simulink model "SVPWMtrials"  (R2015b)
settings: Solver=VariableStepAuto  StartTime=0.0  StopTime=1  RelTol=1e-3
libraries: powerlib x25
(part 3 of 3)

== matlab function SVPWMtrials/Sector2 ==
  data: Sector2 input; Sa1 output; Sa2 output; Sa1P output; Sa2P output; Sb1 output; Sb2 output; Sb1P output; Sb2P output; Sc1 output; Sc2 output; Sc1P output; Sc2P output; rgn2a input; rgn2b input; rgn3 input; rgn4 input; exttime input; Ta input; Tb input; Tc input
function [Sa1, Sa2, Sa1P, Sa2P, Sb1, Sb2, Sb1P, Sb2P, Sc1, Sc2, Sc1P, Sc2P] = fcn(Sector2,rgn2a, rgn2b, rgn3, rgn4,exttime, Ta, Tb, Tc)

Sa1=0; Sa2=0; Sa1P=0; Sa2P=0; Sb1=0; Sb2=0; Sb1P=0; Sb2P=0; Sc1=0; Sc2=0; Sc1P=0; Sc2P=0;
a = exttime;
if(Sector2)
    if(rgn3)
        while(a<exttime+Tc/4)
            Sa1=0; Sa2=1; Sa1P=1; Sa2P=0;
            Sb1=0; Sb2=1; Sb1P=1; Sb2P=0;
            Sc1=0; Sc2=0; Sc1P=1; Sc2P=1;
        a = a+0.000001; %pause(Tc/4);
        end
        while(a<exttime+Tb/2)
            Sa1=0; Sa2=1; Sa1P=1; Sa2P=0;
            Sb1=1; Sb2=1; Sb1P=0; Sb2P=0;
            Sc1=0; Sc2=0; Sc1P=1; Sc2P=1;
            a = a+0.000001; %pause(Tb/2); 
        end
        while(a<exttime+Ta/2)
            Sa1=1; Sa2=1; Sa1P=0; Sa2P=0;
            Sb1=1; Sb2=1; Sb1P=0; Sb2P=0;
            Sc1=0; Sc2=0; Sc1P=1; Sc2P=1;
            a = a+0.000001; %pause(Ta/2); 
        end
        while(a<exttime+Tc/2)
            Sa1=1; Sa2=1; Sa1P=0; Sa2P=0;
            Sb1=1; Sb2=1; Sb1P=0; Sb2P=0;
            Sc1=0; Sc2=1; Sc1P=1; Sc2P=0;       
            a = a+0.000001; %pause(Tc/2);
        end
        while(a<exttime+Ta/2)
            Sa1=1; Sa2=1; Sa1P=0; Sa2P=0;
            Sb1=1; Sb2=1; Sb1P=0; Sb2P=0;
            Sc1=0; Sc2=0; Sc1P=1; Sc2P=1;
            a = a+0.000001; %pause(Ta/2); 
        end
        while(a<exttime+Tb/2)
            Sa1=0; Sa2=1; Sa1P=1; Sa2P=0;
            Sb1=1; Sb2=1; Sb1P=0; Sb2P=0;
            Sc1=0; Sc2=0; Sc1P=1; Sc2P=1;
            a = a+0.000001; %pause(Tb/2); 
        end
        while(a<exttime+Tc/4)
            Sa1=0; Sa2=1; Sa1P=1; Sa2P=0;
            Sb1=0; Sb2=1; Sb1P=1; Sb2P=0;
            Sc1=0; Sc2=0; Sc1P=1; Sc2P=1;
            a = a+0.000001; %pause(Tc/4);       
        end
    end
    
        if(rgn2a)
            while(a<exttime+Tc/4)
                Sa1=0; Sa2=1; Sa1P=1; Sa2P=0;
                Sb1=0; Sb2=1; Sb1P=1; Sb2P=0;
                Sc1=0; Sc2=0; Sc1P=1; Sc2P=1;
                a = a+0.000001; %pause(Tc/4);
            end
            while(a<exttime+Tb/2)
                Sa1=0; Sa2=1; Sa1P=1; Sa2P=0;
                Sb1=1; Sb2=1; Sb1P=0; Sb2P=0;
                Sc1=0; Sc2=0; Sc1P=1; Sc2P=1;
                a = a+0.000001; %pause(Tb/2); 
            end
            while(a<exttime+Ta/2)
                Sa1=0; Sa2=1; Sa1P=1; Sa2P=0;
                Sb1=1; Sb2=1; Sb1P=0; Sb2P=0;
                Sc1=0; Sc2=1; Sc1P=1; Sc2P=0;
                a = a+0.000001; %pause(Ta/2); 
            end
            while(a<exttime+Tc/2)
                Sa1=1; Sa2=1; Sa1P=0; Sa2P=0;
                Sb1=1; Sb2=1; Sb1P=0; Sb2P=0;
                Sc1=0; Sc2=1; Sc1P=1; Sc2P=0;            
                a = a+0.000001; %pause(Tc/2);
            end
            while(a<exttime+Ta/2)
                Sa1=0; Sa2=1; Sa1P=1; Sa2P=0;
                Sb1=1; Sb2=1; Sb1P=0; Sb2P=0;
                Sc1=0; Sc2=1; Sc1P=1; Sc2P=0;
                a = a+0.000001; %pause(Ta/2); 
            end
            while(a<exttime+Tb/2)
                Sa1=0; Sa2=1; Sa1P=1; Sa2P=0;
                Sb1=1; Sb2=1; Sb1P=0; Sb2P=0;
                Sc1=0; Sc2=0; Sc1P=1; Sc2P=1;
                a = a+0.000001; %pause(Tb/2); 
            end
            while(a<exttime+Tc/4)
                Sa1=0; Sa2=1; Sa1P=1; Sa2P=0;
                Sb1=0; Sb2=1; Sb1P=1; Sb2P=0;
                Sc1=0; Sc2=0; Sc1P=1; Sc2P=1;
                a = a+0.000001; %pause(Tc/4);
            end
        end
        if(rgn2b)
            while(a<exttime+Tc/4)
                Sa1=0; Sa2=0; Sa1P=1; Sa2P=1;
                Sb1=0; Sb2=1; Sb1P=1; Sb2P=0;
                Sc1=0; Sc2=0; Sc1P=1; Sc2P=1;
                a = a+0.000001; %pause(Tc/4);
            end
            while(a<exttime+Tb/2)
                Sa1=0; Sa2=1; Sa1P=1; Sa2P=0;
                Sb1=0; Sb2=1; Sb1P=1; Sb2P=0;
                Sc1=0; Sc2=0; Sc1P=1; Sc2P=1;
                a = a+0.000001; %pause(Tb/2); 
            end
            while(a<exttime+Ta/2)
                Sa1=0; Sa2=1; Sa1P=1; Sa2P=0;
                Sb1=1; Sb2=1; Sb1P=0; Sb2P=0;
                Sc1=0; Sc2=0; Sc1P=1; Sc2P=1;
                a = a+0.000001; %pause(Ta/2); 
            end
            while(a<exttime+Tc/2)
                Sa1=0; Sa2=1; Sa1P=1; Sa2P=0;   
                Sb1=1; Sb2=1; Sb1P=0; Sb2P=0;
                Sc1=0; Sc2=1; Sc1P=1; Sc2P=0;
                a = a+0.000001; %pause(Tc/2);
            end
            while(a<exttime+Ta/2)
                Sa1=0; Sa2=1; Sa1P=1; Sa2P=0;
                Sb1=1; Sb2=1; Sb1P=0; Sb2P=0;
                Sc1=0; Sc2=0; Sc1P=1; Sc2P=1;
                a = a+0.000001; %pause(Ta/2); 
            end
            while(a<exttime+Tb/2)
                Sa1=0; Sa2=1; Sa1P=1; Sa2P=0;
                Sb1=0; Sb2=1; Sb1P=1; Sb2P=0;
                Sc1=0; Sc2=0; Sc1P=1; Sc2P=1;
                a = a+0.000001; %pause(Tb/2); 
            end
            while(a<exttime+Tc/4)
                Sa1=0; Sa2=0; Sa1P=1; Sa2P=1;
                Sb1=0; Sb2=1; Sb1P=1; Sb2P=0;
                Sc1=0; Sc2=0; Sc1P=1; Sc2P=1;
                a = a+0.000001; %pause(Tc/4);           
            end
        end    
    if(rgn4)
        while(a<exttime+Tc/4)
            Sa1=0; Sa2=0; Sa1P=1; Sa2P=1;
            Sb1=0; Sb2=1; Sb1P=1; Sb2P=0;
            Sc1=0; Sc2=0; Sc1P=1; Sc2P=1;
            a = a+0.000001; %pause(Tc/4);
        end
        while(a<exttime+Tb/2)
            Sa1=0; Sa2=0; Sa1P=1; Sa2P=1;
            Sb1=1; Sb2=1; Sb1P=0; Sb2P=0;
            Sc1=0; Sc2=0; Sc1P=1; Sc2P=1;
            a = a+0.000001; %pause(Tb/2); 
        end
        while(a<exttime+Ta/2)
            Sa1=0; Sa2=1; Sa1P=1; Sa2P=0;
            Sb1=1; Sb2=1; Sb1P=0; Sb2P=0;
            Sc1=0; Sc2=0; Sc1P=1; Sc2P=1;
            a = a+0.000001; %pause(Ta/2); 
        end
        while(a<exttime+Tc/2)
            Sa1=0; Sa2=1; Sa1P=1; Sa2P=0;
            Sb1=1; Sb2=1; Sb1P=0; Sb2P=0;
            Sc1=0; Sc2=1; Sc1P=1; Sc2P=0;
            a = a+0.000001; %pause(Tc/2); 
        end
        while(a<exttime+Ta/2)
            Sa1=0; Sa2=1; Sa1P=1; Sa2P=0;
            Sb1=1; Sb2=1; Sb1P=0; Sb2P=0;
            Sc1=0; Sc2=0; Sc1P=1; Sc2P=1;
            a = a+0.000001; %pause(Ta/2); 
        end
        while(a<exttime+Tb/2)
            Sa1=0; Sa2=0; Sa1P=1; Sa2P=1;
            Sb1=1; Sb2=1; Sb1P=0; Sb2P=0;
            Sc1=0; Sc2=0; Sc1P=1; Sc2P=1;
            a = a+0.000001; %pause(Tb/2); 
        end
        while(a<exttime+Tc/4)
            Sa1=0; Sa2=0; Sa1P=1; Sa2P=1;
            Sb1=0; Sb2=1; Sb1P=1; Sb2P=0;
            Sc1=0; Sc2=0; Sc1P=1; Sc2P=1;
            a = a+0.000001; %pause(Tc/4);
        end
    end

end

== matlab function SVPWMtrials/Sector3 ==
  data: Sector3 input; Sa1 output; Sa2 output; Sa1P output; Sa2P output; Sb1 output; Sb2 output; Sb1P output; Sb2P output; Sc1 output; Sc2 output; Sc1P output; Sc2P output; rgn2a input; rgn2b input; rgn3 input; rgn4 input; exttime input; Ta input; Tb input; Tc input
function [Sa1, Sa2, Sa1P, Sa2P, Sb1, Sb2, Sb1P, Sb2P, Sc1, Sc2, Sc1P, Sc2P] = fcn(Sector3,rgn2a, rgn2b, rgn3, rgn4,exttime, Ta, Tb, Tc)

Sa1=0; Sa2=0; Sa1P=0; Sa2P=0; Sb1=0; Sb2=0; Sb1P=0; Sb2P=0; Sc1=0; Sc2=0; Sc1P=0; Sc2P=0;
a = exttime;
if(Sector3)
    if(rgn3)
        while(a<exttime+Tc/4)
            Sa1=0; Sa2=0; Sa1P=1; Sa2P=1;
            Sb1=0; Sb2=1; Sb1P=1; Sb2P=0;
            Sc1=0; Sc2=0; Sc1P=1; Sc2P=1;
            a = a+0.000001; %pause(Tc/4);
        end
        while(a<exttime+Tb/2)
            Sa1=0; Sa2=0; Sa1P=1; Sa2P=1;
            Sb1=1; Sb2=1; Sb1P=0; Sb2P=0;
            Sc1=0; Sc2=0; Sc1P=1; Sc2P=1;
            a = a+0.000001; %pause(Tb/2); 
        end
        while(a<exttime+Ta/2)
            Sa1=0; Sa2=0; Sa1P=1; Sa2P=1;
            Sb1=1; Sb2=1; Sb1P=0; Sb2P=0;
            Sc1=0; Sc2=1; Sc1P=1; Sc2P=0;
            a = a+0.000001; %pause(Ta/2); 
        end
        while(a<exttime+Tc/2)
            Sa1=0; Sa2=1; Sa1P=1; Sa2P=0;
            Sb1=1; Sb2=1; Sb1P=0; Sb2P=0;
            Sc1=0; Sc2=1; Sc1P=1; Sc2P=0;
            a = a+0.000001; %pause(Tc/2);
        end
        while(a<exttime+Ta/2)
            Sa1=0; Sa2=0; Sa1P=1; Sa2P=1;
            Sb1=1; Sb2=1; Sb1P=0; Sb2P=0;
            Sc1=0; Sc2=1; Sc1P=1; Sc2P=0;
            a = a+0.000001; %pause(Ta/2); 
        end
        while(a<exttime+Tb/2)
            Sa1=0; Sa2=0; Sa1P=1; Sa2P=1;
            Sb1=1; Sb2=1; Sb1P=0; Sb2P=0;
            Sc1=0; Sc2=0; Sc1P=1; Sc2P=1;
            a = a+0.000001; %pause(Tb/2); 
        end
        while(a<exttime+Tc/4)
            Sa1=0; Sa2=0; Sa1P=1; Sa2P=1;
            Sb1=0; Sb2=1; Sb1P=1; Sb2P=0;
            Sc1=0; Sc2=0; Sc1P=1; Sc2P=1;
            a = a+0.000001; %pause(Tc/4);        
        end
    end

        if(rgn2a)
            while(a<exttime+Tc/4)            
                Sa1=0; Sa2=0; Sa1P=1; Sa2P=1;
                Sb1=0; Sb2=1; Sb1P=1; Sb2P=0;
                Sc1=0; Sc2=0; Sc1P=1; Sc2P=1;
                a = a+0.000001; %pause(Tc/4);
            end
            while(a<exttime+Tb/2)
                Sa1=0; Sa2=0; Sa1P=1; Sa2P=1;
                Sb1=0; Sb2=1; Sb1P=1; Sb2P=0;
                Sc1=0; Sc2=1; Sc1P=1; Sc2P=0;
                a = a+0.000001; %pause(Tb/2); 
            end
            while(a<exttime+Ta/2)
                Sa1=0; Sa2=0; Sa1P=1; Sa2P=1;
                Sb1=1; Sb2=1; Sb1P=0; Sb2P=0;
                Sc1=0; Sc2=1; Sc1P=1; Sc2P=0;
            	a = a+0.000001; %pause(Ta/2); 
            end
            while(a<exttime+Tc/2)
                Sa1=0; Sa2=0; Sa1P=1; Sa2P=1;
                Sb1=1; Sb2=1; Sb1P=0; Sb2P=0;
                Sc1=0; Sc2=0; Sc1P=1; Sc2P=1;
                a = a+0.000001; %pause(Tc/2);
            end
            while(a<exttime+Ta/2)
                Sa1=0; Sa2=0; Sa1P=1; Sa2P=1;
                Sb1=1; Sb2=1; Sb1P=0; Sb2P=0;
                Sc1=0; Sc2=1; Sc1P=1; Sc2P=0;
                a = a+0.000001; %pause(Ta/2); 
            end
            while(a<exttime+Tb/2)
                Sa1=0; Sa2=0; Sa1P=1; Sa2P=1;
                Sb1=0; Sb2=1; Sb1P=1; Sb2P=0;
                Sc1=0; Sc2=1; Sc1P=1; Sc2P=0;
                a = a+0.000001; %pause(Tb/2); 
            end
            while(a<exttime+Tc/4)
                Sa1=0; Sa2=0; Sa1P=1; Sa2P=1;
                Sb1=0; Sb2=1; Sb1P=1; Sb2P=0;
                Sc1=0; Sc2=0; Sc1P=1; Sc2P=1;
                a = a+0.000001; %pause(Tc/4); 
            end
        end
        if(rgn2b)
            while(a<exttime+Tc/4)
                Sa1=0; Sa2=0; Sa1P=1; Sa2P=1;
                Sb1=0; Sb2=1; Sb1P=1; Sb2P=0;
                Sc1=0; Sc2=1; Sc1P=1; Sc2P=0;
                a = a+0.000001; %pause(Tc/4);
            end
            while(a<exttime+Tb/2)
                Sa1=0; Sa2=0; Sa1P=1; Sa2P=1;
                Sb1=1; Sb2=1; Sb1P=0; Sb2P=0;
                Sc1=0; Sc2=1; Sc1P=1; Sc2P=0;
                a = a+0.000001; %pause(Tb/2); 
            end
            while(a<exttime+Ta/2)
                Sa1=0; Sa2=1; Sa1P=1; Sa2P=0;
                Sb1=1; Sb2=1; Sb1P=0; Sb2P=0;
                Sc1=0; Sc2=1; Sc1P=1; Sc2P=0;
                a = a+0.000001; %pause(Ta/2); 
            end
            while(a<exttime+Tc/2)
                Sa1=0; Sa2=1; Sa1P=1; Sa2P=0;
                Sb1=1; Sb2=1; Sb1P=0; Sb2P=0;
                Sc1=1; Sc2=1; Sc1P=0; Sc2P=0;
                a = a+0.000001; %pause(Tc/2);
            end
            while(a<exttime+Ta/2)
                Sa1=0; Sa2=1; Sa1P=1; Sa2P=0;
                Sb1=1; Sb2=1; Sb1P=0; Sb2P=0;
                Sc1=0; Sc2=1; Sc1P=1; Sc2P=0;
                a = a+0.000001; %pause(Ta/2); 
            end
            while(a<exttime+Tb/2)
                Sa1=0; Sa2=0; Sa1P=1; Sa2P=1;
                Sb1=1; Sb2=1; Sb1P=0; Sb2P=0;
                Sc1=0; Sc2=1; Sc1P=1; Sc2P=0;
                a = a+0.000001; %pause(Tb/2); 
            end
            while(a<exttime+Tc/4)
                Sa1=0; Sa2=0; Sa1P=1; Sa2P=1;
                Sb1=0; Sb2=1; Sb1P=1; Sb2P=0;
                Sc1=0; Sc2=1; Sc1P=1; Sc2P=0;
                a = a+0.000001; %pause(Tc/4);            
            end
        end

    if(rgn4)
        while(a<exttime+Tc/4)
            Sa1=0; Sa2=0; Sa1P=1; Sa2P=1;
            Sb1=0; Sb2=1; Sb1P=1; Sb2P=0;
            Sc1=0; Sc2=1; Sc1P=1; Sc2P=0;
            a = a+0.000001; %pause(Tc/4);
        end
        while(a<exttime+Tb/2)
            Sa1=0; Sa2=0; Sa1P=1; Sa2P=1;
            Sb1=1; Sb2=1; Sb1P=0; Sb2P=0;
            Sc1=0; Sc2=1; Sc1P=1; Sc2P=0;
            a = a+0.000001; %pause(Tb/2); 
        end
        while(a<exttime+Ta/2)
            Sa1=0; Sa2=0; Sa1P=1; Sa2P=1;
            Sb1=1; Sb2=1; Sb1P=0; Sb2P=0;
            Sc1=1; Sc2=1; Sc1P=0; Sc2P=0;
            a = a+0.000001; %pause(Ta/2); 
        end
        while(a<exttime+Tc/2)
            Sa1=0; Sa2=1; Sa1P=1; Sa2P=0;
            Sb1=1; Sb2=1; Sb1P=0; Sb2P=0;
            Sc1=1; Sc2=1; Sc1P=0; Sc2P=0;
            a = a+0.000001; %pause(Tc/2);
        end
        while(a<exttime+Ta/2)
            Sa1=0; Sa2=0; Sa1P=1; Sa2P=1;
            Sb1=1; Sb2=1; Sb1P=0; Sb2P=0;
            Sc1=1; Sc2=1; Sc1P=0; Sc2P=0;
            a = a+0.000001; %pause(Ta/2); 
        end
        while(a<exttime+Tb/2)
            Sa1=0; Sa2=0; Sa1P=1; Sa2P=1;
            Sb1=1; Sb2=1; Sb1P=0; Sb2P=0;
            Sc1=0; Sc2=1; Sc1P=1; Sc2P=0;
            a = a+0.000001; %pause(Tb/2); 
        end
        while(a<exttime+Tc/4)
            Sa1=0; Sa2=0; Sa1P=1; Sa2P=1;
            Sb1=0; Sb2=1; Sb1P=1; Sb2P=0;
            Sc1=0; Sc2=1; Sc1P=1; Sc2P=0;
            a = a+0.000001; %pause(Tc/4);
        end
    end
end

== matlab function SVPWMtrials/Sector4 ==
  data: Sector4 input; Sa1 output; Sa2 output; Sa1P output; Sa2P output; Sb1 output; Sb2 output; Sb1P output; Sb2P output; Sc1 output; Sc2 output; Sc1P output; Sc2P output; rgn2a input; rgn2b input; rgn3 input; rgn4 input; exttime input; Ta input; Tb input; Tc input
function [Sa1, Sa2, Sa1P, Sa2P, Sb1, Sb2, Sb1P, Sb2P, Sc1, Sc2, Sc1P, Sc2P] = fcn(Sector4,rgn2a, rgn2b, rgn3, rgn4,exttime, Ta, Tb, Tc)

Sa1=0; Sa2=0; Sa1P=0; Sa2P=0; Sb1=0; Sb2=0; Sb1P=0; Sb2P=0; Sc1=0; Sc2=0; Sc1P=0; Sc2P=0;
a = exttime;
if(Sector4)
    if(rgn3) 
        while(a<exttime+Tc/4)
            Sa1=0; Sa2=1; Sa1P=1; Sa2P=0;
            Sb1=1; Sb2=1; Sb1P=0; Sb2P=0;
            Sc1=1; Sc2=1; Sc1P=0; Sc2P=0;
            a = a+0.000001; %pause(Tc/4);
        end
        while(a<exttime+Tb/2)
            Sa1=0; Sa2=0; Sa1P=1; Sa2P=1;
            Sb1=1; Sb2=1; Sb1P=0; Sb2P=0;
            Sc1=1; Sc2=1; Sc1P=0; Sc2P=0;
            a = a+0.000001; %pause(Tb/2); 
        end
        while(a<exttime+Ta/2)
            Sa1=0; Sa2=0; Sa1P=1; Sa2P=1;
            Sb1=0; Sb2=1; Sb1P=1; Sb2P=0;
            Sc1=1; Sc2=1; Sc1P=0; Sc2P=0;
            a = a+0.000001; %pause(Ta/2); 
        end
        while(a<exttime+Tc/2)
            Sa1=0; Sa2=0; Sa1P=1; Sa2P=1;
            Sb1=0; Sb2=1; Sb1P=1; Sb2P=0;
            Sc1=0; Sc2=1; Sc1P=1; Sc2P=0;
            a = a+0.000001; %pause(Tc/2);
        end
        while(a<exttime+Ta/2)
            Sa1=0; Sa2=0; Sa1P=1; Sa2P=1;
            Sb1=0; Sb2=1; Sb1P=1; Sb2P=0;
            Sc1=1; Sc2=1; Sc1P=0; Sc2P=0;
            a = a+0.000001; %pause(Ta/2); 
        end
        while(a<exttime+Tb/2)
            Sa1=0; Sa2=0; Sa1P=1; Sa2P=1;
            Sb1=1; Sb2=1; Sb1P=0; Sb2P=0;
            Sc1=1; Sc2=1; Sc1P=0; Sc2P=0;
            a = a+0.000001; %pause(Tb/2); 
        end
        while(a<exttime+Tc/4)
            Sa1=0; Sa2=1; Sa1P=1; Sa2P=0;
            Sb1=1; Sb2=1; Sb1P=0; Sb2P=0;
            Sc1=1; Sc2=1; Sc1P=0; Sc2P=0;
            a = a+0.000001; %pause(Tc/4);
        end
    end
        if(rgn2a)
            while(a<exttime+Tc/4)
                Sa1=0; Sa2=1; Sa1P=1; Sa2P=0;
                Sb1=1; Sb2=1; Sb1P=0; Sb2P=0;
                Sc1=1; Sc2=1; Sc1P=0; Sc2P=0;
                a = a+0.000001; %pause(Tc/4);
            end
            while(a<exttime+Tb/2)
                Sa1=0; Sa2=1; Sa1P=1; Sa2P=0;
                Sb1=0; Sb2=1; Sb1P=1; Sb2P=0;
                Sc1=1; Sc2=1; Sc1P=0; Sc2P=0;
                a = a+0.000001; %pause(Tb/2); 
            end
            while(a<exttime+Ta/2)
                Sa1=0; Sa2=0; Sa1P=1; Sa2P=1;
                Sb1=0; Sb2=1; Sb1P=1; Sb2P=0;
                Sc1=1; Sc2=1; Sc1P=0; Sc2P=0;
                a = a+0.000001; %pause(Ta/2); 
            end
            while(a<exttime+Tc/2)
                Sa1=0; Sa2=0; Sa1P=1; Sa2P=1;
                Sb1=0; Sb2=1; Sb1P=1; Sb2P=0;
                Sc1=0; Sc2=1; Sc1P=1; Sc2P=0;
                a = a+0.000001; %pause(Tc/2);
            end
            while(a<exttime+Ta/2)
                Sa1=0; Sa2=0; Sa1P=1; Sa2P=1;
                Sb1=0; Sb2=1; Sb1P=1; Sb2P=0;
                Sc1=1; Sc2=1; Sc1P=0; Sc2P=0;
                a = a+0.000001; %pause(Ta/2); 
            end
            while(a<exttime+Tb/2)
                Sa1=0; Sa2=1; Sa1P=1; Sa2P=0;
                Sb1=0; Sb2=1; Sb1P=1; Sb2P=0;
                Sc1=1; Sc2=1; Sc1P=0; Sc2P=0;
                a = a+0.000001; %pause(Tb/2); 
            end
            while(a<exttime+Tc/4)
                Sa1=0; Sa2=1; Sa1P=1; Sa2P=0;
                Sb1=1; Sb2=1; Sb1P=0; Sb2P=0;
                Sc1=1; Sc2=1; Sc1P=0; Sc2P=0;
                a = a+0.000001; %pause(Tc/4);           
            end
        end
        if(rgn2b)
            while(a<exttime+Tc/4)
                Sa1=0; Sa2=1; Sa1P=1; Sa2P=0;
                Sb1=0; Sb2=1; Sb1P=1; Sb2P=0;
                Sc1=1; Sc2=1; Sc1P=0; Sc2P=0;
                a = a+0.000001; %pause(Tc/4);
            end
            while(a<exttime+Tb/2)
                Sa1=0; Sa2=0; Sa1P=1; Sa2P=1;
                Sb1=0; Sb2=1; Sb1P=1; Sb2P=0;
                Sc1=1; Sc2=1; Sc1P=0; Sc2P=0;
            a = a+0.000001; %pause(Tb/2); 
            end
            while(a<exttime+Ta/2)
                Sa1=0; Sa2=0; Sa1P=1; Sa2P=1;
                Sb1=0; Sb2=1; Sb1P=1; Sb2P=0;
                Sc1=0; Sc2=1; Sc1P=1; Sc2P=0;
                a = a+0.000001; %pause(Ta/2); 
            end
            while(a<exttime+Tc/2)
                Sa1=0; Sa2=0; Sa1P=1; Sa2P=1;
                Sb1=0; Sb2=0; Sb1P=1; Sb2P=1;
                Sc1=0; Sc2=1; Sc1P=1; Sc2P=0;
                a = a+0.000001; %pause(Tc/2);
            end
            while(a<exttime+Ta/2)
                Sa1=0; Sa2=0; Sa1P=1; Sa2P=1;
                Sb1=0; Sb2=1; Sb1P=1; Sb2P=0;
                Sc1=0; Sc2=1; Sc1P=1; Sc2P=0;
                a = a+0.000001; %pause(Ta/2); 
            end
            while(a<exttime+Tb/2)
                Sa1=0; Sa2=0; Sa1P=1; Sa2P=1;
                Sb1=0; Sb2=1; Sb1P=1; Sb2P=0;
                Sc1=1; Sc2=1; Sc1P=0; Sc2P=0;
                a = a+0.000001; %pause(Tb/2); 
            end
            while(a<exttime+Tc/4)
                Sa1=0; Sa2=1; Sa1P=1; Sa2P=0;
                Sb1=0; Sb2=1; Sb1P=1; Sb2P=0;
                Sc1=1; Sc2=1; Sc1P=0; Sc2P=0;
                a = a+0.000001; %pause(Tc/4);                      
            end
        end
    if(rgn4)
        while(a<exttime+Tc/4)
            Sa1=0; Sa2=1; Sa1P=1; Sa2P=0;
            Sb1=0; Sb2=1; Sb1P=1; Sb2P=0;
            Sc1=1; Sc2=1; Sc1P=0; Sc2P=0;
            a = a+0.000001; %pause(Tc/4);
        end
        while(a<exttime+Tb/2)
            Sa1=0; Sa2=0; Sa1P=1; Sa2P=1;
            Sb1=0; Sb2=1; Sb1P=1; Sb2P=0;
            Sc1=1; Sc2=1; Sc1P=0; Sc2P=0;
            a = a+0.000001; %pause(Tb/2); 
        end
        while(a<exttime+Ta/2)
            Sa1=0; Sa2=0; Sa1P=1; Sa2P=1;
            Sb1=0; Sb2=0; Sb1P=1; Sb2P=1;
            Sc1=1; Sc2=1; Sc1P=0; Sc2P=0;
            a = a+0.000001; %pause(Ta/2); 
        end
        while(a<exttime+Tc/2)
            Sa1=0; Sa2=0; Sa1P=1; Sa2P=1;
            Sb1=0; Sb2=0; Sb1P=1; Sb2P=1;
            Sc1=0; Sc2=1; Sc1P=1; Sc2P=0;
            a = a+0.000001; %pause(Tc/2);
        end
        while(a<exttime+Ta/2)
            Sa1=0; Sa2=0; Sa1P=1; Sa2P=1;
            Sb1=0; Sb2=0; Sb1P=1; Sb2P=1;
            Sc1=1; Sc2=1; Sc1P=0; Sc2P=0;
            a = a+0.000001; %pause(Ta/2); 
        end
        while(a<exttime+Tb/2)
            Sa1=0; Sa2=0; Sa1P=1; Sa2P=1;
            Sb1=0; Sb2=1; Sb1P=1; Sb2P=0;
            Sc1=1; Sc2=1; Sc1P=0; Sc2P=0;
            a = a+0.000001; %pause(Tb/2); 
        end
        while(a<exttime+Tc/4)
            Sa1=0; Sa2=1; Sa1P=1; Sa2P=0;
            Sb1=0; Sb2=1; Sb1P=1; Sb2P=0;
            Sc1=1; Sc2=1; Sc1P=0; Sc2P=0;
            a = a+0.000001; %pause(Tc/4);
        end
    end     
end
end

== matlab function SVPWMtrials/Sector5 ==
  data: Sector5 input; Sa1 output; Sa2 output; Sa1P output; Sa2P output; Sb1 output; Sb2 output; Sb1P output; Sb2P output; Sc1 output; Sc2 output; Sc1P output; Sc2P output; rgn2a input; rgn2b input; rgn3 input; rgn4 input; exttime input; Ta input; Tb input; Tc input
function [Sa1, Sa2, Sa1P, Sa2P, Sb1, Sb2, Sb1P, Sb2P, Sc1, Sc2, Sc1P, Sc2P] = fcn(Sector5,rgn2a, rgn2b, rgn3, rgn4,exttime, Ta, Tb, Tc)

Sa1=0; Sa2=0; Sa1P=0; Sa2P=0; Sb1=0; Sb2=0; Sb1P=0; Sb2P=0; Sc1=0; Sc2=0; Sc1P=0; Sc2P=0;
a = exttime;
if(Sector5)
    if(rgn3)
        while(a<exttime+Tc/4)
            Sa1=0; Sa2=1; Sa1P=1; Sa2P=0;
            Sb1=0; Sb2=1; Sb1P=1; Sb2P=0;
            Sc1=1; Sc2=1; Sc1P=0; Sc2P=0;
            a = a+0.000001; %pause(Tc/4);
        end
        while(a<exttime+Tb/2)
            Sa1=0; Sa2=1; Sa1P=1; Sa2P=0;
            Sb1=0; Sb2=0; Sb1P=1; Sb2P=1;
            Sc1=1; Sc2=1; Sc1P=0; Sc2P=0;
            a = a+0.000001; %pause(Tb/2); 
        end
        while(a<exttime+Ta/2)
            Sa1=0; Sa2=0; Sa1P=1; Sa2P=1;
            Sb1=0; Sb2=0; Sb1P=1; Sb2P=1;
            Sc1=1; Sc2=1; Sc1P=0; Sc2P=0;
            a = a+0.000001; %pause(Ta/2); 
        end
        while(a<exttime+Tc/2)
            Sa1=0; Sa2=0; Sa1P=1; Sa2P=1;
            Sb1=0; Sb2=0; Sb1P=1; Sb2P=1;
            Sc1=0; Sc2=1; Sc1P=1; Sc2P=0;
            a = a+0.000001; %pause(Tc/2);
        end
        while(a<exttime+Ta/2)
            Sa1=0; Sa2=0; Sa1P=1; Sa2P=1;
            Sb1=0; Sb2=0; Sb1P=1; Sb2P=1;
            Sc1=1; Sc2=1; Sc1P=0; Sc2P=0;
            a = a+0.000001; %pause(Ta/2); 
        end
        while(a<exttime+Tb/2)
            Sa1=0; Sa2=1; Sa1P=1; Sa2P=0;
            Sb1=0; Sb2=0; Sb1P=1; Sb2P=1;
            Sc1=1; Sc2=1; Sc1P=0; Sc2P=0;
            a = a+0.000001; %pause(Tb/2); 
        end
        while(a<exttime+Tc/4)
            Sa1=0; Sa2=1; Sa1P=1; Sa2P=0;
            Sb1=0; Sb2=1; Sb1P=1; Sb2P=0;
            Sc1=1; Sc2=1; Sc1P=0; Sc2P=0;
            a = a+0.000001; %pause(Tc/4);
        end
    end
        if(rgn2a)
            while(a<exttime+Tc/4)
                Sa1=0; Sa2=1; Sa1P=1; Sa2P=0;
                Sb1=0; Sb2=1; Sb1P=1; Sb2P=0;
                Sc1=1; Sc2=1; Sc1P=0; Sc2P=0;
                a = a+0.000001; %pause(Tc/4);
            end
            while(a<exttime+Tb/2)
                Sa1=0; Sa2=1; Sa1P=1; Sa2P=0;
                Sb1=0; Sb2=0; Sb1P=1; Sb2P=1;
                Sc1=1; Sc2=1; Sc1P=0; Sc2P=0;
                a = a+0.000001; %pause(Tb/2); 
            end
            while(a<exttime+Ta/2)
                Sa1=0; Sa2=1; Sa1P=1; Sa2P=0;
                Sb1=0; Sb2=0; Sb1P=1; Sb2P=1;
                Sc1=0; Sc2=1; Sc1P=1; Sc2P=0;        
                a = a+0.000001; %pause(Ta/2); 
            end
            while(a<exttime+Tc/2)
                Sa1=0; Sa2=0; Sa1P=1; Sa2P=1;
                Sb1=0; Sb2=0; Sb1P=1; Sb2P=1;
                Sc1=0; Sc2=1; Sc1P=1; Sc2P=0;
                a = a+0.000001; %pause(Tc/2);
            end
            while(a<exttime+Ta/2)
                Sa1=0; Sa2=1; Sa1P=1; Sa2P=0;
                Sb1=0; Sb2=0; Sb1P=1; Sb2P=1;
                Sc1=0; Sc2=1; Sc1P=1; Sc2P=0;        
                a = a+0.000001; %pause(Ta/2); 
            end
            while(a<exttime+Tb/2)
                Sa1=0; Sa2=1; Sa1P=1; Sa2P=0;
                Sb1=0; Sb2=0; Sb1P=1; Sb2P=1;
                Sc1=1; Sc2=1; Sc1P=0; Sc2P=0;
                a = a+0.000001; %pause(Tb/2); 
            end
            while(a<exttime+Tc/4)
                Sa1=0; Sa2=1; Sa1P=1; Sa2P=0;
                Sb1=0; Sb2=1; Sb1P=1; Sb2P=0;
                Sc1=1; Sc2=1; Sc1P=0; Sc2P=0;
                a = a+0.000001;%pause(Tc/4);
            end
        end
        if(rgn2b)
            while(a<exttime+Tc/4)
                Sa1=1; Sa2=1; Sa1P=0; Sa2P=0;
                Sb1=0; Sb2=1; Sb1P=1; Sb2P=0;
                Sc1=1; Sc2=1; Sc1P=0; Sc2P=0;
                a = a+0.000001; %pause(Tc/4);
            end
            while(a<exttime+Tb/2)
                Sa1=0; Sa2=1; Sa1P=1; Sa2P=0;
                Sb1=0; Sb2=1; Sb1P=1; Sb2P=0;
                Sc1=1; Sc2=1; Sc1P=0; Sc2P=0;
                a = a+0.000001; %pause(Tb/2); 
            end
            while(a<exttime+Ta/2)
                Sa1=0; Sa2=1; Sa1P=1; Sa2P=0;
                Sb1=0; Sb2=0; Sb1P=1; Sb2P=1;
                Sc1=1; Sc2=1; Sc1P=0; Sc2P=0;
                a = a+0.000001; %pause(Ta/2); 
            end
            while(a<exttime+Tc/2)
                Sa1=0; Sa2=1; Sa1P=1; Sa2P=0;
                Sb1=0; Sb2=0; Sb1P=1; Sb2P=1;
                Sc1=0; Sc2=1; Sc1P=1; Sc2P=0;
                a = a+0.000001; %pause(Tc/2);
            end
            while(a<exttime+Ta/2)
                Sa1=0; Sa2=1; Sa1P=1; Sa2P=0;
                Sb1=0; Sb2=0; Sb1P=1; Sb2P=1;
                Sc1=1; Sc2=1; Sc1P=0; Sc2P=0;
                a = a+0.000001; %pause(Ta/2); 
            end
            while(a<exttime+Tb/2)
                Sa1=0; Sa2=1; Sa1P=1; Sa2P=0;
                Sb1=0; Sb2=1; Sb1P=1; Sb2P=0;
                Sc1=1; Sc2=1; Sc1P=0; Sc2P=0;
                a = a+0.000001; %pause(Tb/2); 
            end
            while(a<exttime+Tc/4)
                Sa1=1; Sa2=1; Sa1P=0; Sa2P=0;
                Sb1=0; Sb2=1; Sb1P=1; Sb2P=0;
                Sc1=1; Sc2=1; Sc1P=0; Sc2P=0;
                a = a+0.000001; %pause(Tc/4);               
            end
        end
    if(rgn4)
        while(a<exttime+Tc/4)
            Sa1=1; Sa2=1; Sa1P=0; Sa2P=0; 
            Sb1=0; Sb2=1; Sb1P=1; Sb2P=0;
            Sc1=1; Sc2=1; Sc1P=0; Sc2P=0;
            a = a+0.000001; %pause(Tc/4);
        end
        while(a<exttime+Tb/2)
            Sa1=1; Sa2=1; Sa1P=0; Sa2P=0;
            Sb1=0; Sb2=0; Sb1P=1; Sb2P=1;
            Sc1=1; Sc2=1; Sc1P=0; Sc2P=0;
            a = a+0.000001; %pause(Tb/2); 
        end
        while(a<exttime+Ta/2)
            Sa1=0; Sa2=1; Sa1P=1; Sa2P=0;
            Sb1=0; Sb2=0; Sb1P=1; Sb2P=1;
            Sc1=1; Sc2=1; Sc1P=0; Sc2P=0;
            a = a+0.000001; %pause(Ta/2); 
        end
        while(a<exttime+Tc/2)
            Sa1=0; Sa2=1; Sa1P=1; Sa2P=0;
            Sb1=0; Sb2=0; Sb1P=1; Sb2P=1;
            Sc1=0; Sc2=1; Sc1P=1; Sc2P=0;
            a = a+0.000001; %pause(Tc/2);
        end
        while(a<exttime+Ta/2)
            Sa1=0; Sa2=1; Sa1P=1; Sa2P=0;
            Sb1=0; Sb2=0; Sb1P=1; Sb2P=1;
            Sc1=1; Sc2=1; Sc1P=0; Sc2P=0;
            a = a+0.000001; %pause(Ta/2); 
        end
        while(a<exttime+Tb/2)
            Sa1=1; Sa2=1; Sa1P=0; Sa2P=0;
            Sb1=0; Sb2=0; Sb1P=1; Sb2P=1;
            Sc1=1; Sc2=1; Sc1P=0; Sc2P=0;
            a = a+0.000001; %pause(Tb/2); 
        end
        while(a<exttime+Tc/4)
            Sa1=1; Sa2=1; Sa1P=0; Sa2P=0; 
            Sb1=0; Sb2=1; Sb1P=1; Sb2P=0;
            Sc1=1; Sc2=1; Sc1P=0; Sc2P=0;
            a = a+0.000001; %pause(Tc/4);
        end
    end
    
end

== matlab function SVPWMtrials/Sector6 ==
  data: Sector6 input; Sa1 output; Sa2 output; Sa1P output; Sa2P output; Sb1 output; Sb2 output; Sb1P output; Sb2P output; Sc1 output; Sc2 output; Sc1P output; Sc2P output; rgn2a input; rgn2b input; rgn3 input; rgn4 input; exttime input; Ta input; Tb input; Tc input
function [Sa1, Sa2, Sa1P, Sa2P, Sb1, Sb2, Sb1P, Sb2P, Sc1, Sc2, Sc1P, Sc2P] = fcn(Sector6,rgn2a, rgn2b, rgn3, rgn4,exttime, Ta, Tb, Tc)

Sa1=0; Sa2=0; Sa1P=0; Sa2P=0; Sb1=0; Sb2=0; Sb1P=0; Sb2P=0; Sc1=0; Sc2=0; Sc1P=0; Sc2P=0;
a = exttime;
if(Sector6)
    if(rgn3)
        while(a<exttime+Tc/4)
            Sa1=1; Sa2=1; Sa1P=0; Sa2P=0;
            Sb1=0; Sb2=1; Sb1P=1; Sb2P=0;
            Sc1=1; Sc2=1; Sc1P=0; Sc2P=0;
            a = a+0.000001; %pause(Tc/4);
        end
        while(a<exttime+Tb/2)
            Sa1=1; Sa2=1; Sa1P=0; Sa2P=0;
            Sb1=0; Sb2=0; Sb1P=1; Sb2P=1;
            Sc1=1; Sc2=1; Sc1P=0; Sc2P=0;
            a = a+0.000001; %pause(Tb/2); 
        end
        while(a<exttime+Ta/2)
            Sa1=1; Sa2=1; Sa1P=0; Sa2P=0;
            Sb1=0; Sb2=0; Sb1P=1; Sb2P=1;
            Sc1=0; Sc2=1; Sc1P=1; Sc2P=0;
            a = a+0.000001; %pause(Ta/2); 
        end
        while(a<exttime+Tc/2)
            Sa1=0; Sa2=1; Sa1P=1; Sa2P=0;
            Sb1=0; Sb2=0; Sb1P=1; Sb2P=1;
            Sc1=0; Sc2=1; Sc1P=1; Sc2P=0;
            a = a+0.000001; %pause(Tc/2);
        end
        while(a<exttime+Ta/2)
            Sa1=1; Sa2=1; Sa1P=0; Sa2P=0;
            Sb1=0; Sb2=0; Sb1P=1; Sb2P=1;
            Sc1=0; Sc2=1; Sc1P=1; Sc2P=0;
            a = a+0.000001; %pause(Ta/2); 
        end
        while(a<exttime+Tb/2)
            Sa1=1; Sa2=1; Sa1P=0; Sa2P=0;
            Sb1=0; Sb2=0; Sb1P=1; Sb2P=1;
            Sc1=1; Sc2=1; Sc1P=0; Sc2P=0;
            a = a+0.000001; %pause(Tb/2); 
        end
        while(a<exttime+Tc/4)
            Sa1=1; Sa2=1; Sa1P=0; Sa2P=0;
            Sb1=0; Sb2=1; Sb1P=1; Sb2P=0;
            Sc1=1; Sc2=1; Sc1P=0; Sc2P=0;
            a = a+0.000001; %pause(Tc/4);
        end
    end
        if(rgn2a)
            while(a<exttime+Tc/4)
                Sa1=1; Sa2=1; Sa1P=0; Sa2P=0;
                Sb1=0; Sb2=1; Sb1P=1; Sb2P=0;
                Sc1=1; Sc2=1; Sc1P=0; Sc2P=0;
                a = a+0.000001; %pause(Tc/4);
            end
            while(a<exttime+Tb/2)
                Sa1=1; Sa2=1; Sa1P=0; Sa2P=0;
                Sb1=0; Sb2=1; Sb1P=1; Sb2P=0;
                Sc1=0; Sc2=1; Sc1P=1; Sc2P=0;
                a = a+0.000001; %pause(Tb/2); 
            end
            while(a<exttime+Ta/2)
                Sa1=1; Sa2=1; Sa1P=0; Sa2P=0;
                Sb1=0; Sb2=0; Sb1P=1; Sb2P=1;
                Sc1=0; Sc2=1; Sc1P=1; Sc2P=0;
                a = a+0.000001; %pause(Ta/2); 
            end
            while(a<exttime+Tc/2)
                Sa1=0; Sa2=1; Sa1P=1; Sa2P=0;
                Sb1=0; Sb2=0; Sb1P=1; Sb2P=1;
                Sc1=0; Sc2=1; Sc1P=1; Sc2P=0;
                a = a+0.000001; %pause(Tc/2);
            end
            while(a<exttime+Ta/2)
                Sa1=1; Sa2=1; Sa1P=0; Sa2P=0;
                Sb1=0; Sb2=0; Sb1P=1; Sb2P=1;
                Sc1=0; Sc2=1; Sc1P=1; Sc2P=0;
                a = a+0.000001; %pause(Ta/2); 
            end
            while(a<exttime+Tb/2)
                Sa1=1; Sa2=1; Sa1P=0; Sa2P=0;
                Sb1=0; Sb2=1; Sb1P=1; Sb2P=0;
                Sc1=0; Sc2=1; Sc1P=1; Sc2P=0;
                a = a+0.000001; %pause(Tb/2);  
            end
            while(a<exttime+Tc/4)
                Sa1=1; Sa2=1; Sa1P=0; Sa2P=0;
                Sb1=0; Sb2=1; Sb1P=1; Sb2P=0;
                Sc1=1; Sc2=1; Sc1P=0; Sc2P=0;
                a = a+0.000001; %pause(Tc/4);
            end
        end
        if(rgn2b)
            while(a<exttime+Tc/4)
                Sa1=1; Sa2=1; Sa1P=0; Sa2P=0;
                Sb1=0; Sb2=1; Sb1P=1; Sb2P=0;
                Sc1=0; Sc2=1; Sc1P=1; Sc2P=0;
                a = a+0.000001; %pause(Tc/4);
            end
            while(a<exttime+Tb/2)
                Sa1=1; Sa2=1; Sa1P=0; Sa2P=0;
                Sb1=0; Sb2=0; Sb1P=1; Sb2P=1;
                Sc1=0; Sc2=1; Sc1P=1; Sc2P=0;
                a = a+0.000001; %pause(Tb/2); 
            end
            while(a<exttime+Ta/2)
                Sa1=0; Sa2=1; Sa1P=1; Sa2P=0;
                Sb1=0; Sb2=0; Sb1P=1; Sb2P=1;
                Sc1=0; Sc2=1; Sc1P=1; Sc2P=0;
                a = a+0.000001; %pause(Ta/2); 
            end
            while(a<exttime+Tc/2)
                Sa1=0; Sa2=1; Sa1P=1; Sa2P=0;
                Sb1=0; Sb2=0; Sb1P=1; Sb2P=1;
                Sc1=0; Sc2=0; Sc1P=1; Sc2P=1;
                a = a+0.000001; %pause(Tc/2);
            end
            while(a<exttime+Ta/2)
                Sa1=0; Sa2=1; Sa1P=1; Sa2P=0;
                Sb1=0; Sb2=0; Sb1P=1; Sb2P=1;
                Sc1=0; Sc2=1; Sc1P=1; Sc2P=0;
                a = a+0.000001; %pause(Ta/2); 
            end
            while(a<exttime+Tb/2)
                Sa1=1; Sa2=1; Sa1P=0; Sa2P=0;
                Sb1=0; Sb2=0; Sb1P=1; Sb2P=1;
                Sc1=0; Sc2=1; Sc1P=1; Sc2P=0;
                a = a+0.000001; %pause(Tb/2); 
            end
            while(a<exttime+Tc/4)
                Sa1=1; Sa2=1; Sa1P=0; Sa2P=0;
                Sb1=0; Sb2=1; Sb1P=1; Sb2P=0;
                Sc1=0; Sc2=1; Sc1P=1; Sc2P=0;
                a = a+0.000001; %pause(Tc/4);
            end
        end
    if(rgn4)
        while(a<exttime+Tc/4)
            Sa1=1; Sa2=1; Sa1P=0; Sa2P=0;
            Sb1=0; Sb2=1; Sb1P=1; Sb2P=0;
            Sc1=0; Sc2=1; Sc1P=1; Sc2P=0;
            a = a+0.000001; %pause(Tc/4);
        end
        while(a<exttime+Tb/2)
            Sa1=1; Sa2=1; Sa1P=0; Sa2P=0;
            Sb1=0; Sb2=0; Sb1P=1; Sb2P=1;
            Sc1=0; Sc2=1; Sc1P=1; Sc2P=0;
            a = a+0.000001; %pause(Tb/2); 
        end
        while(a<exttime+Ta/2)
            Sa1=1; Sa2=1; Sa1P=0; Sa2P=0;
            Sb1=0; Sb2=0; Sb1P=1; Sb2P=1;
            Sc1=0; Sc2=0; Sc1P=1; Sc2P=1;
            a = a+0.000001; %pause(Ta/2); 
        end
        while(a<exttime+Tc/2)
            Sa1=0; Sa2=1; Sa1P=1; Sa2P=0;
            Sb1=0; Sb2=0; Sb1P=1; Sb2P=1;
            Sc1=0; Sc2=0; Sc1P=1; Sc2P=1;
            a = a+0.000001; %pause(Tc/2);
        end
        while(a<exttime+Ta/2)
            Sa1=1; Sa2=1; Sa1P=0; Sa2P=0;
            Sb1=0; Sb2=0; Sb1P=1; Sb2P=1;
            Sc1=0; Sc2=0; Sc1P=1; Sc2P=1;
            a = a+0.000001; %pause(Ta/2); 
        end
        while(a<exttime+Tb/2)
            Sa1=1; Sa2=1; Sa1P=0; Sa2P=0;
            Sb1=0; Sb2=0; Sb1P=1; Sb2P=1;
            Sc1=0; Sc2=1; Sc1P=1; Sc2P=0;
            a = a+0.000001; %pause(Tb/2);  
        end
        while(a<exttime+Tc/4)
            Sa1=1; Sa2=1; Sa1P=0; Sa2P=0;
            Sb1=0; Sb2=1; Sb1P=1; Sb2P=0;
            Sc1=0; Sc2=1; Sc1P=1; Sc2P=0;
            a = a+0.000001; %pause(Tc/4);
        end
    end
end
